simulink model "rad_to_rpm"  (R2020a)
settings: Solver=VariableStepAuto  StartTime=0.0  StopTime=10.0  MaxStep=.01  RelTol=1e-3
settings Model: Creator=Administrator  LastModifiedBy=Administrator

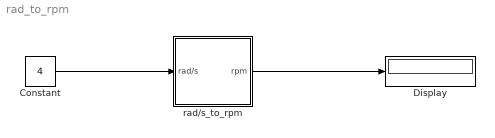
== system rad_to_rpm ==
  Constant : Constant  Value=4
  Display : Display
  rad/s_to_rpm : Subsystem
  wires:
  Constant/1 -> rad/s_to_rpm/1(rad/s)
  rad/s_to_rpm/1(rpm) -> Display/1

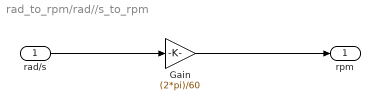
== system rad_to_rpm/rad//s_to_rpm ==
  rad/s : Inport
  Gain : Gain  Gain=(2*pi)/60
  rpm : Outport
  wires:
  Gain/1 -> rpm/1
  rad/s/1 -> Gain/1
